simulink model "PlantaHinf_Simulacion"  (R2016a)
settings: Solver=VariableStepAuto  StartTime=0.0  StopTime=10  RelTol=1e-3
undefined symbols (not defined in the file or in its folder): K1
settings Model: Creator=Julián  LastModifiedBy=i95sa
settings DataIOCC: LimitDataPoints=on  SaveFormat=Array  SignalLoggingSaveFormat=ModelDataLogs
settings DebuggingCC: SolverPrmCheckMsg=warning  MultiTaskDSMMsg=warning  MultiTaskCondExecSysMsg=none
settings HardwareCC: ProdBitPerPointer=32  ProdLargestAtomicFloat=None  ProdIntDivRoundTo=Undefined  ProdEndianess=Unspecified  ProdWordSize=32  ProdHWDeviceType=32-bit Generic
settings ModelReferenceCC: PropagateSignalLabelsOutOfModel=off
settings ConfigComp: CovModelRefEnable=Off

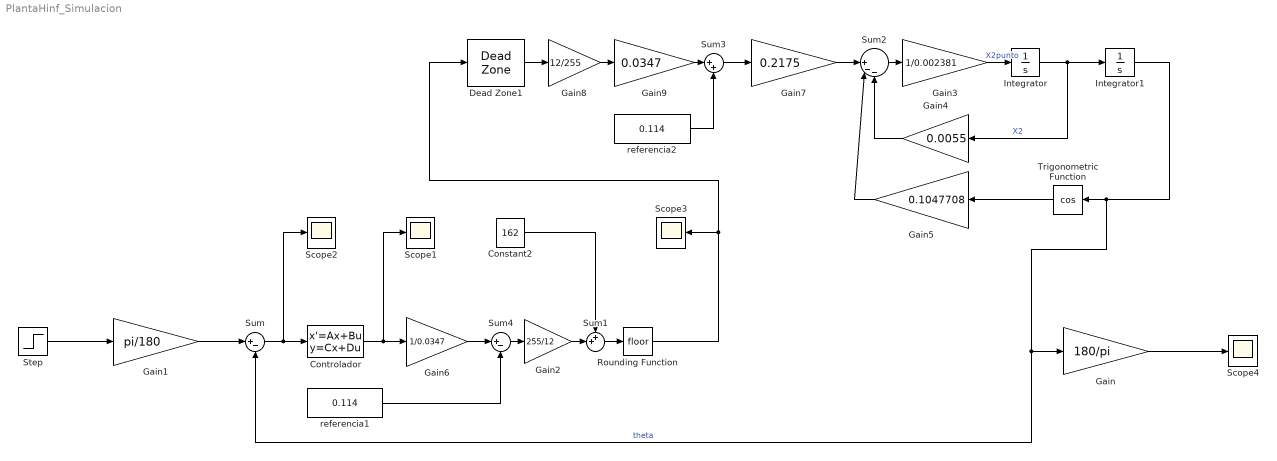
== system PlantaHinf_Simulacion ==
  Constant2 : Constant  Value=162
  Controlador : StateSpace  A=K1.a  B=K1.b  C=K1.c  D=K1.d  X0=0
  Dead Zone1 : DeadZone  LowerValue=0  UpperValue=0  SaturateOnIntegerOverflow=on
  Gain : Gain  Gain=180/pi
  Gain1 : Gain  Gain=pi/180
  Gain2 : Gain  Gain=255/12
  Gain3 : Gain  Gain=1/0.002381
  Gain4 : Gain  Gain=0.0055
  Gain5 : Gain  Gain=0.1047708
  Gain6 : Gain  Gain=1/0.0347
  Gain7 : Gain  Gain=0.2175
  Gain8 : Gain  Gain=12/255
  Gain9 : Gain  Gain=0.0347
  Integrator : Integrator
  Integrator1 : Integrator
  Rounding Function : Rounding
  Scope{1..4} (4 alike) : Scope
  Step : Step  Time=0  After=0  SampleTime=0
  Sum : Sum  Inputs=|+-
  Sum1 : Sum  Inputs=++|
  Sum2 : Sum  Inputs=||+--
  Sum3 : Sum  Inputs=|++
  Sum4 : Sum  Inputs=|+-
  Trigonometric Function : Trigonometry  Operator=cos
  referencia1 : Constant  Value=0.114
  referencia2 : Constant  Value=0.114
  wires:
  Step/1 -> Gain1/1
  Sum/1 -> Controlador/1, Scope2/1
  Controlador/1 -> Scope1/1, Gain6/1
  Gain/1 -> Scope4/1
  Gain1/1 -> Sum/1
  referencia1/1 -> Sum4/2
  Sum4/1 -> Gain2/1
  Sum1/1 -> Rounding Function/1
  Constant2/1 -> Sum1/1
  Gain2/1 -> Sum1/2
  Gain6/1 -> Sum4/1
  Sum2/1 -> Gain3/1
  Gain3/1 -> Integrator/1  "X2punto"
  Integrator/1 -> Integrator1/1, Gain4/1  "X2"
  Trigonometric Function/1 -> Gain5/1
  Gain4/1 -> Sum2/3
  Integrator1/1 -> Gain/1, Sum/2, Trigonometric Function/1  "theta"
  Gain5/1 -> Sum2/2
  Gain7/1 -> Sum2/1
  referencia2/1 -> Sum3/2
  Sum3/1 -> Gain7/1
  Gain8/1 -> Gain9/1
  Gain9/1 -> Sum3/1
  Dead Zone1/1 -> Gain8/1
  Rounding Function/1 -> Dead Zone1/1, Scope3/1
